simulink model "FIR_SymmetricDecimatorStream_Ex3"  (R2024a)
settings: Solver=VariableStepAuto  StartTime=0.0  StopTime=8192/100e3  RelTol=1e-3
PostLoadFcn:
  | Fs = 100000;  % Sampling Frequency
  | Fpass = 5000;              % Passband Frequency
  | Fstop = 10000;             % Stopband Frequency
  | Dpass = 0.0046051376314;   % Passband Ripple
  | Dstop = 0.00025118864315;  % Stopband Attenuation
  | dens  = 16;                % Density Factor
  | % Calculate the order from the parameters using FIRPMORD.
  | [N, Fo, Ao, W] = firpmord([Fpass, Fstop]/(Fs/2), [1 0], [Dpass, Dstop]);
  | % Calculate the coefficients using the FIRPM function.
  | coeffs = firpm(N, Fo, Ao, W, {dens});
  | AIE_Coeffs = (int16(coeffs(1:32)*2^15));
undefined symbols (not defined in the file): firpmord, None, S, vsva2197, xcvc1902
libraries: aieUtilities x4, dspsrcs4 x2, aieDSP x1, dspmlti4 x1, vmcUtilities x1
settings Model: Creator=sdegala  LastModifiedBy=sdegala
settings ModelReferenceCC: EnableRefExpFcnMdlSchedulingChecks=on
settings RTWCC: GPUComputeCapability=3.5

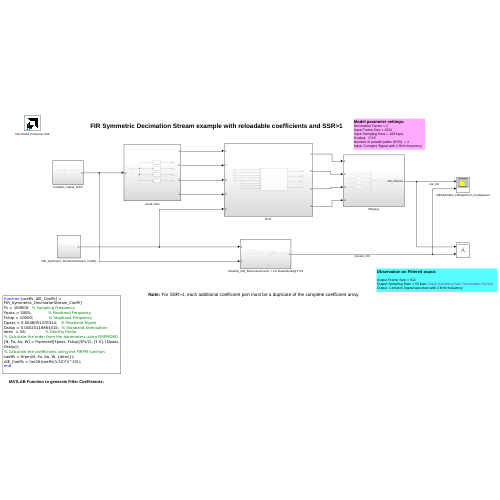
[thumbnail: Simulink's stored preview of the top-level diagram]
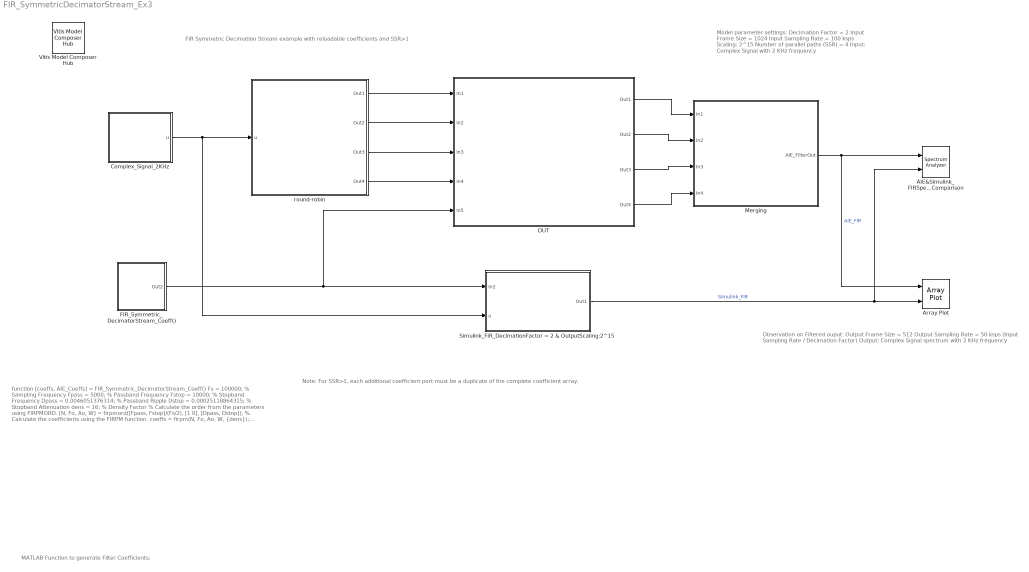
== system FIR_SymmetricDecimatorStream_Ex3 ==
  note: Note: For SSR>1, each additional coefficient port must be a duplicate of the complete coefficient array.
  note: FIR Symmetric Decimation Stream example with reloadable coefficients and SSR>1
  note: Model parameter settings:
      | Decimation Factor = 2
      | Input Frame Size = 1024
      | Input Sampling Rate = 100 ksps
      | Scaling: 2^15
      | Number of parallel paths (SSR) = 4
      | Input: Complex Signal with 2 KHz frequency
  note: Observation on Filtered ouput:
      |
      | Output Frame Size = 512
      | Output Sampling Rate = 50 ksps (Input Sampling Rate / Decimation Factor)
      | Output: Complex Signal spectrum with 2 KHz frequency
  note: function [coeffs, AIE_Coeffs] = FIR_Symmetric_DecimatorStream_Coeff()
      | Fs = 100000; % Sampling Frequency
      | Fpass = 5000; % Passband Frequency
      | Fstop = 10000; % Stopband Frequency
      | Dpass = 0.0046051376314; % Passband Ripple
      | Dstop = 0.00025118864315; % Stopband Attenuation
      | dens = 16; % Density Factor
      | % Calculate the order from the parameters using FIRPMORD.
      | [N, Fo, Ao, W] = firpmord([Fpass, Fstop]/(Fs/2), [1 0], [Dpass, Dstop]);
      | % Calculate the coefficients using the FIRPM function.
      | coeffs = firpm(N, Fo, Ao, W, {dens});
      | AIE_Coeffs = (int16(coeffs(1:32)*2^15));
      | end
  note: MATLAB Function to generate Filter Coefficients:
  AIE&Simulink_FIRSpectrum_Comparison : SpectrumAnalyzer  NumInputPorts=2  WindowPosition=[530.000000,85.000000,1280.000000,600.000000,]  Visible=on  ScopeFrameLocation=window  SampleRate=50000  Span=49999.99999999999  StartFrequency=-24999.999999999996  StopFrequency=24999.999999999996  AveragingMethod=Exponential  YLimits=[33.2677,123.2864]  ShowLegend=on  AllowFFTLengthLessThanSamplesPerUpdate=on  DefaultConfigurationName=spbscopes.SpectrumAnalyzerBlockCfg  IsFrequencyInputMode=0  FrequencyVectorPort=0  FrequencyVectorFromPort=0  FrequencyInputRBWPort=0  FrequencyInputRBWFromPort=0
  Array Plot : ArrayPlot  NumInputPorts=2  WindowPosition=[585.000000,453.000000,800.000000,500.000000,]  Visible=on  ScopeFrameLocation=window  PlotType=Line  YLimits=[-21674.125 21597.125]  ShowLegend=on
  Complex_Signal_2KHz : Subsystem
  DUT : Subsystem
  FIR_Symmetric_DecimatorStream_Coeff() : Subsystem
  Merging : Subsystem
  Simulink_FIR_DecimationFactor = 2 & OutputScaling:2^15 : Subsystem
  Vitis Model Composer Hub : vmcUtilities/Vitis Model Composer Hub  Tag=genX  CodeGeneration=off  StartColumn=1  NumberOfColumns=1  TargetDirectory=./code  exportDesign=off  analyzeDesign=off  validateDesignOnHw=off  ExportType=AI Engines  IpVendor=xilinx.com  IpLibrary=hls  IpVersion=1.0  IpHWLanguage=Verilog  AieCompilerOptions={}  AieSimulatorOptions={}  CreateTestbench=off  TestbenchStackSize=10  RunRtlSim=off  RunCSim=off  RunAieSim=off  AieSimTimeout=50000  RunAieSimProfiling=off  LaunchVitisAnalyzer=off  PlotOutput=off  RunX86Sim=off  X86SimTimeout=10  GenHwImage=off  GenLibadfXo=off  GenHwValidationCode=off  PlatformType=Not Specified  HwSystemType=Baremetal  HwValidationTarget=hw  ProjDevice=xcvc1902-vsva2197-1LP-e-S  ProjDevicePart=xcvc1902-vsva2197-1LP-e-S  AIEType=AIE  SamplePeriod=-1  ClockFrequency=200  DataPathParallelism=1  xilinxfamily=versalaicore  part=xcvc1902  speed=-1LP-e-S  package=vsva2197  directory=./netlist  testbench=off  incr_netlist=off  synthesis_tool=Vivado  clock_wrapper=Clock Enables  dbl_ovrd=According to Block Masks  dcm_input_clock_period=10  sysclk_period=10  simulink_period=1  eval_field=0  LogFileName=''  NThreads=4
  round-robin : Subsystem
  wires:
  Complex_Signal_2KHz/1(u) -> Simulink_FIR_DecimationFactor = 2 & OutputScaling:2^15/2(u), round-robin/1(u)
  Merging/1(AIE_FilterOut) -> Array Plot/1, AIE&Simulink_FIRSpectrum_Comparison/1  "AIE_FIR"
  Simulink_FIR_DecimationFactor = 2 & OutputScaling:2^15/1(Out1) -> AIE&Simulink_FIRSpectrum_Comparison/2, Array Plot/2  "Simulink_FIR"
  FIR_Symmetric_DecimatorStream_Coeff()/1(Out2) -> DUT/5(In5), Simulink_FIR_DecimationFactor = 2 & OutputScaling:2^15/1(In2)
  round-robin/1(Out1) -> DUT/1(In1)
  round-robin/2(Out2) -> DUT/2(In2)
  round-robin/3(Out3) -> DUT/3(In3)
  round-robin/4(Out4) -> DUT/4(In4)
  DUT/1(Out1) -> Merging/1(In1)
  DUT/2(Out2) -> Merging/2(In2)
  DUT/3(Out3) -> Merging/3(In3)
  DUT/4(Out4) -> Merging/4(In4)

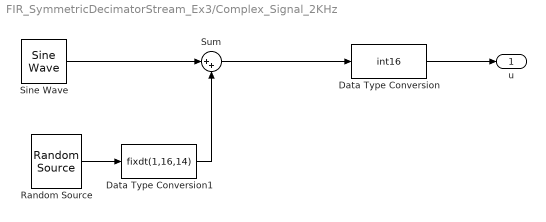
== system FIR_SymmetricDecimatorStream_Ex3/Complex_Signal_2KHz ==
  Data Type Conversion : DataTypeConversion  OutMin=[-1]  OutMax=[1]  OutDataTypeStr=int16  ConvertRealWorld=Stored Integer (SI)  SaturateOnIntegerOverflow=off  RndMeth=Floor
  Data Type Conversion1 : DataTypeConversion  OutDataTypeStr=fixdt(1,16,14)  SaturateOnIntegerOverflow=off  RndMeth=Floor
  Random Source : dspsrcs4/Random Source  SrcType=Gaussian  MinVal=0  MaxVal=1  MeanVal=0  VarVal=1e-6  RepMode=Specify seed  rawSeed=1  IsInherit=off  SampTime=1/100e3  SampFrame=1024  OutComplex=Complex  DataType=single  SimulateUsing=Interpreted execution
  Sine Wave : dspsrcs4/Sine Wave  Amplitude=1  Frequency=2e3  Phase=0  SampleMode=Discrete  OutComplex=Complex  CompMethod=Table lookup  TableSize=Speed  SampleTime=1/100e3  SamplesPerFrame=1024  ResetState=Restart at time zero  OutputFrames=off  dataType=Fixed-point  wordLen=16  udDataType=sfix(16)  fracBitsMode=User-defined  numFracBits=14  OutDataTypeStr=fixdt(1,16,14)  LastOutDataTypeStr=fixdt(1,16,14)
  Sum : Sum  Inputs=|++
  u : Outport
  wires:
  Data Type Conversion/1 -> u/1
  Sine Wave/1 -> Sum/1
  Sum/1 -> Data Type Conversion/1
  Random Source/1 -> Data Type Conversion1/1
  Data Type Conversion1/1 -> Sum/2

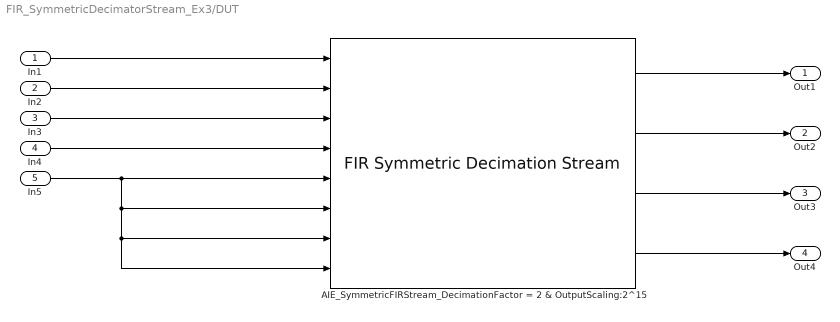
== system FIR_SymmetricDecimatorStream_Ex3/DUT ==
  In1 : Inport
  In2 : Inport  Port=2
  In3 : Inport  Port=3
  In4 : Inport  Port=4
  In5 : Inport  Port=5
  "AIE_SymmetricFIRStream_DecimationFactor = 2 & OutputScaling:2^15 " : aieDSP/FIR Symmetric Decimation Stream  data_type=cint16  coef_type=int16  use_coeff_reload=on  dual_ip=off  num_outputs=off  coeff=AIE_Coeffs  fir_length=64  decimate_factor=2  input_window_size=1024  shift_val=15  rnd_mode=Ceiling  sat_mode=0-None  ssr=4  casc_length=2  AIE_VARIANT=1  TP_API=1  blockJsonConstraints=[]  blockJsonConstraintsInternal=[]  spec=vmc_stream_fir_decimate_sym.json  SerializedMaskParamNames=[]  SerializedMaskParamValues=[]  SerializedMaskParamVisibilities=[]  block_type=FIR Symmetric Decimation Stream  SerializedMaskParamDataypes=typename|typename|uint|uint|uint|coef_type|uint|uint|uint|uint|uint|uint|uint|uint|uint|uint  SerializedMaskParamEnumStrArr=0|0|0|0|0|0|0|0|0|0|Floor,Ceiling,Round to positive infinity,Round to negative infinity,Round symmetrical to infinity,Round symmetrical to zero,Round convergent to even,Round convergent to odd|0-None,1-Asymmetric,3-Symmetric|0|0|0|0  SerializedMaskParamEnumValArr=0|0|0|0|0|0|0|0|0|0|0,1,2,3,4,5,6,7|0,1,3|0|0|0|0  SerializedMaskParamVectorArr=0|0|0|0|0|1|0|0|0|0|0|0|0|0|0|0  SerializedMaskParamKeys=TT_DATA|TT_COEFF|TP_USE_COEFF_RELOAD|TP_DUAL_IP|TP_NUM_OUTPUTS|coeff|TP_FIR_LEN|TP_DECIMATE_FACTOR|TP_INPUT_WINDOW_VSIZE|TP_SHIFT|TP_RND|TP_SAT|TP_SSR|TP_CASC_LEN|AIE_VARIANT|TP_API
  Out1 : Outport
  Out2 : Outport  Port=2
  Out3 : Outport  Port=3
  Out4 : Outport  Port=4
  wires:
  "AIE_SymmetricFIRStream_DecimationFactor = 2 & OutputScaling:2^15 "/1 -> Out1/1
  "AIE_SymmetricFIRStream_DecimationFactor = 2 & OutputScaling:2^15 "/2 -> Out2/1
  In3/1 -> "AIE_SymmetricFIRStream_DecimationFactor = 2 & OutputScaling:2^15 "/3
  "AIE_SymmetricFIRStream_DecimationFactor = 2 & OutputScaling:2^15 "/3 -> Out3/1
  "AIE_SymmetricFIRStream_DecimationFactor = 2 & OutputScaling:2^15 "/4 -> Out4/1
  In2/1 -> "AIE_SymmetricFIRStream_DecimationFactor = 2 & OutputScaling:2^15 "/2
  In1/1 -> "AIE_SymmetricFIRStream_DecimationFactor = 2 & OutputScaling:2^15 "/1
  In4/1 -> "AIE_SymmetricFIRStream_DecimationFactor = 2 & OutputScaling:2^15 "/4
  In5/1 -> "AIE_SymmetricFIRStream_DecimationFactor = 2 & OutputScaling:2^15 "/8, "AIE_SymmetricFIRStream_DecimationFactor = 2 & OutputScaling:2^15 "/7, "AIE_SymmetricFIRStream_DecimationFactor = 2 & OutputScaling:2^15 "/6, "AIE_SymmetricFIRStream_DecimationFactor = 2 & OutputScaling:2^15 "/5

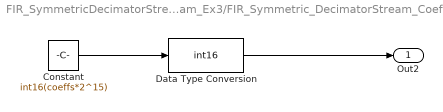
== system FIR_SymmetricDecimatorStream_Ex3/FIR_Symmetric_DecimatorStream_Coeff() ==
  Constant : Constant  Value=int16(coeffs*2^15)
  Data Type Conversion : DataTypeConversion  OutMin=[-1]  OutMax=[1]  OutDataTypeStr=int16  ConvertRealWorld=Stored Integer (SI)  SaturateOnIntegerOverflow=off  RndMeth=Floor
  Out2 : Outport
  wires:
  Constant/1 -> Data Type Conversion/1
  Data Type Conversion/1 -> Out2/1

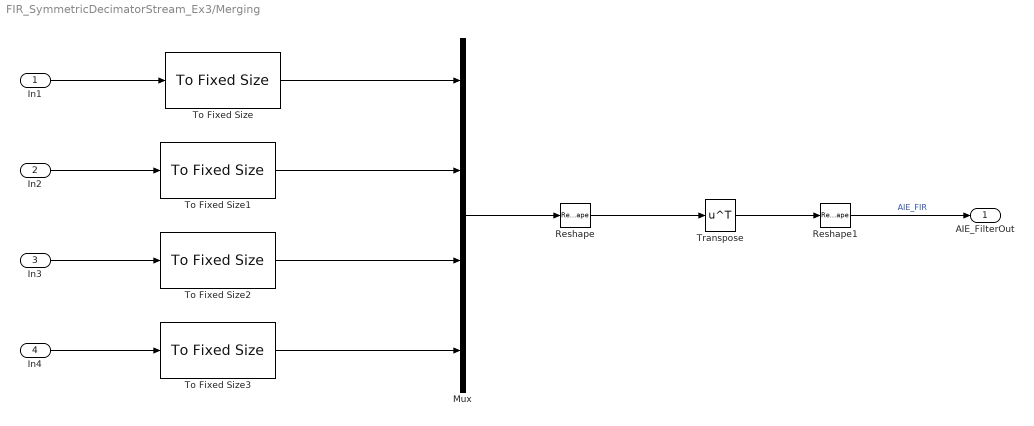
== system FIR_SymmetricDecimatorStream_Ex3/Merging ==
  In1 : Inport
  In2 : Inport  Port=2
  In3 : Inport  Port=3
  In4 : Inport  Port=4
  Mux : Mux
  Reshape : Reshape  OutputDimensionality=Customize  OutputDimensions=[128, 4]
  Reshape1 : Reshape  OutputDimensions=[1, 10]
  To Fixed Size{,1..3} (4 alike) : aieUtilities/To Fixed Size  Mode=Stop simulation when input variable-size signal is not full  OutputSize=Inherit: Same as input  CopyMethod=Buffer samples to form output  HasStatusOutput=on
  Transpose : Math  Operator=transpose
  AIE_FilterOut : Outport
  wires:
  Reshape/1 -> Transpose/1
  To Fixed Size1/1 -> Mux/2
  In2/1 -> To Fixed Size1/1
  Transpose/1 -> Reshape1/1
  To Fixed Size/1 -> Mux/1
  Mux/1 -> Reshape/1
  Reshape1/1 -> AIE_FilterOut/1  "AIE_FIR"
  In1/1 -> To Fixed Size/1
  In4/1 -> To Fixed Size3/1
  To Fixed Size3/1 -> Mux/4
  In3/1 -> To Fixed Size2/1
  To Fixed Size2/1 -> Mux/3

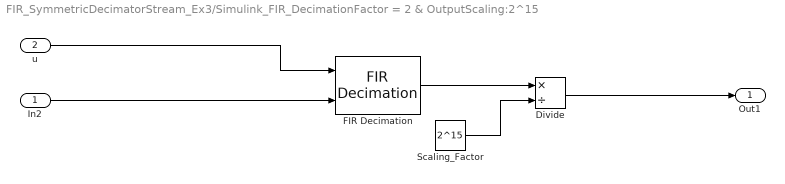
== system FIR_SymmetricDecimatorStream_Ex3/Simulink_FIR_DecimationFactor = 2 & OutputScaling:2^15 ==
  In2 : Inport
  u : Inport  Port=2
  Divide : Product  Inputs=*/  OutDataTypeStr=int16
  FIR Decimation : dspmlti4/FIR Decimation  FilterSource=Input port  h=int16(firpm(63, [0;0.1;0.2;1], [1;1;0;0], [1;18.3333831245308], {16})*2^15)  D=2  filtStruct=Direct form  FilterObject=firpmord([5e3, 10e3]/(100e3/2), [1 0], [0.0046051376314, 0.0001995262315])  InputProcessing=Columns as channels (frame based)  framing=Enforce single-rate processing  AllowArbitraryInputLength=off  inputOffset=0  outputBufInitCond=0  roundingMode=Floor  overflowMode=off  firstCoeffDataTypeStr=Inherit: Same word length as input  firstCoeffMin=[]  firstCoeffMax=[]  firstCoeffLastDataTypeStr=Inherit: Same word length as input  prodOutputMode=Binary point scaling  prodOutputWordLength=32  prodOutputFracLength=0  prodOutputDataTypeStr=fixdt(1,32,0)  prodOutputLastDataTypeStr=fixdt(1,32,0)  accumMode=Binary point scaling  accumWordLength=48  accumFracLength=0  accumDataTypeStr=fixdt(1,48,0)  accumLastDataTypeStr=fixdt(1,48,0)  outputDataTypeStr=Inherit: Same as product output  outputMin=[]  outputMax=[]  outputLastDataTypeStr=Inherit: Same as product output
  Scaling_Factor : Constant  Value=2^15  OutDataTypeStr=int32
  Out1 : Outport
  wires:
  Scaling_Factor/1 -> Divide/2
  FIR Decimation/1 -> Divide/1
  u/1 -> FIR Decimation/1
  Divide/1 -> Out1/1
  In2/1 -> FIR Decimation/2

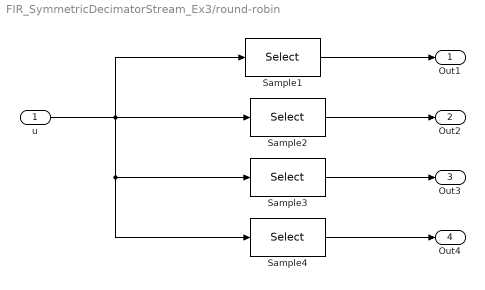
== system FIR_SymmetricDecimatorStream_Ex3/round-robin ==
  u : Inport
  Sample1 : Selector  InputPortWidth=1024  IndexOptions=Index vector (dialog)  Indices=1:4:1024  OutputSizes=1
  Sample2 : Selector  InputPortWidth=1024  IndexOptions=Index vector (dialog)  Indices=2:4:1024  OutputSizes=1
  Sample3 : Selector  InputPortWidth=1024  IndexOptions=Index vector (dialog)  Indices=3:4:1024  OutputSizes=1
  Sample4 : Selector  InputPortWidth=1024  IndexOptions=Index vector (dialog)  Indices=4:4:1024  OutputSizes=1
  Out1 : Outport
  Out2 : Outport  Port=2
  Out3 : Outport  Port=3
  Out4 : Outport  Port=4
  wires:
  u/1 -> Sample4/1, Sample3/1, Sample2/1, Sample1/1
  Sample2/1 -> Out2/1
  Sample1/1 -> Out1/1
  Sample3/1 -> Out3/1
  Sample4/1 -> Out4/1
